simulink library "carterlib"  (R2023a)
settings: Solver=VariableStepAuto  StartTime=0.0  StopTime=10.0  RelTol=1e-3
libraries: arduinolib x6, simulink x1
settings Model: Creator=kawata  LastModifiedBy=kawata
settings RTWCC: GPUComputeCapability=5.0

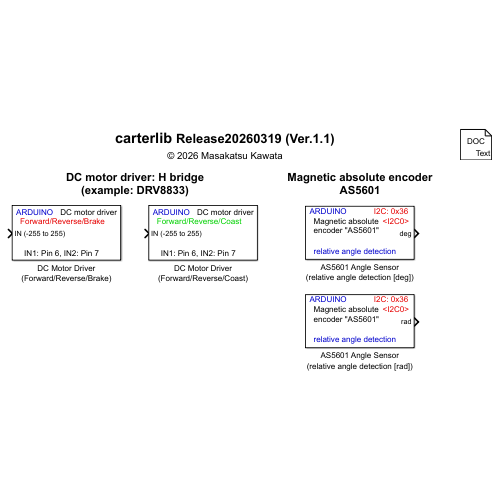
[thumbnail: Simulink's stored preview of the top-level diagram]
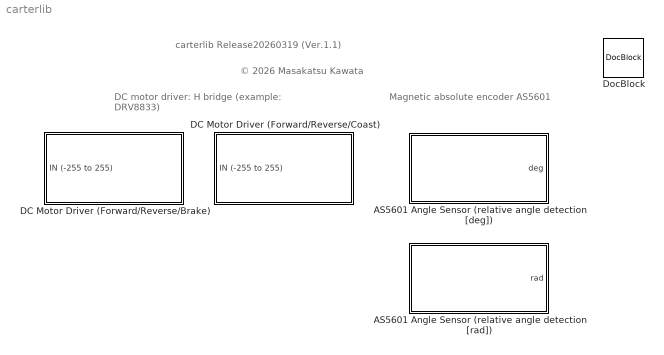
== system carterlib ==
  note: DC motor driver: H bridge
      | (example: DRV8833)
  note: Magnetic absolute encoder
      | AS5601
  note: carterlib Release20260319 (Ver.1.1)
  note: © 2026 Masakatsu Kawata
  AS5601 Angle Sensor (relative angle detection [deg]) : Subsystem  mask{sample_time=-1, I2CModule=0}
      mask prompts: sample_time "Sample Time (-1 for inherited)"; I2CModule "I2C Module"
      mask TypeOptions I2CModule: I2C Read (0x0E: ANGLE)/I2CModule
      mask DialogControl ParameterGroupVar Prompt: パラメーター
      mask Display:
      | color('blue');
      | text(5,60,'ARDUINO')
      | 
      | color('black');
      | text(10,48,'Magnetic absolute')
      | text(10,36,'encoder "AS5601"')
      | 
      | color('blue');
      | text(10, 10, 'relative angle detection');
      | 
      | color('red');
      | text(85, 60, 'I2C: 0x36');
      | 
      | color('red');
      | module = get_param(gcb, 'I2CModule');
      | text(96, 48, ['<I2C' module '>']);
  AS5601 Angle Sensor (relative angle detection [rad]) : Subsystem  mask{sample_time=-1, I2CModule=0}
      mask prompts: sample_time "Sample Time (-1 for inherited)"; I2CModule "I2C Module"
      mask TypeOptions I2CModule: I2C Read (0x0E: ANGLE)/I2CModule
      mask DialogControl ParameterGroupVar Prompt: パラメーター
      mask Display:
      | color('blue');
      | text(5,60,'ARDUINO')
      | 
      | color('black');
      | text(10,48,'Magnetic absolute')
      | text(10,36,'encoder "AS5601"')
      | 
      | color('blue');
      | text(10, 10, 'relative angle detection');
      | 
      | color('red');
      | text(85, 60, 'I2C: 0x36');
      | 
      | color('red');
      | module = get_param(gcb, 'I2CModule');
      | text(96, 48, ['<I2C' module '>']);
  DC Motor Driver (Forward/Reverse/Brake) : Subsystem  mask(Forward/Reverse/Brake){IN1pin=6, IN2pin=7}
      mask prompts: IN1pin "Pin Number (IN1)"; IN2pin "Pin Number (IN2)"
      mask help:
      | IN: -255 to +255
      | ---------------------------------
      | Example
      |
      |   [Arduino MEGA 2560]
      |     Pin Number: 2-13, 44-46
      |
      |   [Arduino UNO R3]
      |     Pin Number: 3, 5, 6, 9-11
      | ---------------------------------
      mask DialogControl ParameterGroupVar Prompt: パラメーター
      mask Display:
      | color('blue');
      | text(5,60,'ARDUINO')
      | 
      | color('black');
      | text(60,60,'DC motor driver')
      | 
      | color('red');
      | text(10,48,['Forward/Reverse/Brake'])
      | 
      | color('black');
      | text(15,8,['IN1: Pin ' num2str(IN1pin) ', IN2: Pin ' num2str(IN2pin)])
  DC Motor Driver (Forward/Reverse/Coast) : Subsystem  mask(Forward/Reverse/Coast){IN1pin=6, IN2pin=7}
      mask prompts: IN1pin "Pin Number (IN1)"; IN2pin "Pin Number (IN2)"
      mask help:
      | IN: -255 to +255
      | ---------------------------------
      | Example
      |
      |   [Arduino MEGA 2560]
      |     Pin Number: 2-13, 44-46
      |
      |   [Arduino UNO R3]
      |     Pin Number: 3, 5, 6, 9-11
      | ---------------------------------
      mask DialogControl ParameterGroupVar Prompt: パラメーター
      mask Display:
      | color('blue');
      | text(5,60,'ARDUINO')
      | 
      | color('black');
      | text(60,60,'DC motor driver')
      | 
      | color('green');
      | text(10,48,'Forward/Reverse/Coast')
      | 
      | color('black');
      | text(15,8,['IN1: Pin ' num2str(IN1pin) ...
      |          ', IN2: Pin ' num2str(IN2pin)])
  DocBlock : simulink/Model-Wide Utilities/DocBlock  DocumentType=Text
      content=|
      | carterlib Ver.1.0
      | Copyright (c) 2026 Masakatsu Kawata
      | Released under the MIT License.
      | See LICENSE for details.

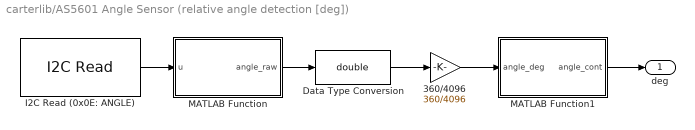
== system carterlib/AS5601 Angle Sensor (relative angle detection [deg]) ==
  360/4096 : Gain  Gain=360/4096
  Data Type Conversion : DataTypeConversion  OutDataTypeStr=double  SaturateOnIntegerOverflow=off  RndMeth=Floor
  I2C Read (0x0E: ANGLE) : arduinolib/I2C Read  I2CModule=0  Mode=Master  SlaveAddress=0x36  SlaveByteOrder=LittleEndian  Direction=Receiver  RegisterAddressMode=on  RegisterAddress=0x0E  SlaveDataType=uint8  DataLength=2  NoAck=off  RepeatedStart=off  OutputStatus=off  blockPlatform=ARDUINO  SampleTime=sample_time
  MATLAB Function : MATLAB Function  TreatAsAtomicUnit=on
  MATLAB Function1 : MATLAB Function  TreatAsAtomicUnit=on
  deg : Outport
  wires:
  MATLAB Function/1(angle_raw) -> Data Type Conversion/1
  360/4096/1 -> MATLAB Function1/1(angle_deg)
  I2C Read (0x0E: ANGLE)/1 -> MATLAB Function/1(u)
  Data Type Conversion/1 -> 360/4096/1
  MATLAB Function1/1(angle_cont) -> deg/1

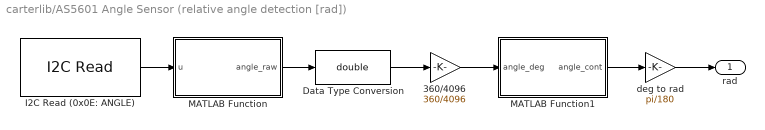
== system carterlib/AS5601 Angle Sensor (relative angle detection [rad]) ==
  360/4096 : Gain  Gain=360/4096
  Data Type Conversion : DataTypeConversion  OutDataTypeStr=double  SaturateOnIntegerOverflow=off  RndMeth=Floor
  I2C Read (0x0E: ANGLE) : arduinolib/I2C Read  I2CModule=0  Mode=Master  SlaveAddress=0x36  SlaveByteOrder=LittleEndian  Direction=Receiver  RegisterAddressMode=on  RegisterAddress=0x0E  SlaveDataType=uint8  DataLength=2  NoAck=off  RepeatedStart=off  OutputStatus=off  blockPlatform=ARDUINO  SampleTime=sample_time
  MATLAB Function : MATLAB Function  TreatAsAtomicUnit=on
  MATLAB Function1 : MATLAB Function  TreatAsAtomicUnit=on
  deg to rad : Gain  Gain=pi/180
  rad : Outport
  wires:
  MATLAB Function1/1(angle_cont) -> deg to rad/1
  Data Type Conversion/1 -> 360/4096/1
  I2C Read (0x0E: ANGLE)/1 -> MATLAB Function/1(u)
  360/4096/1 -> MATLAB Function1/1(angle_deg)
  MATLAB Function/1(angle_raw) -> Data Type Conversion/1
  deg to rad/1 -> rad/1

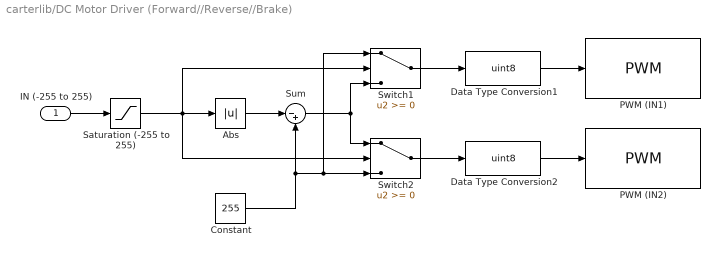
== system carterlib/DC Motor Driver (Forward//Reverse//Brake) ==
  IN (-255 to 255) : Inport
  Abs : Abs  SaturateOnIntegerOverflow=off
  Constant : Constant  Value=255  SampleTime=-1
  Data Type Conversion1 : DataTypeConversion  OutDataTypeStr=uint8  SaturateOnIntegerOverflow=off  RndMeth=Floor
  Data Type Conversion2 : DataTypeConversion  OutDataTypeStr=uint8  SaturateOnIntegerOverflow=off  RndMeth=Floor
  PWM (IN1) : arduinolib/PWM  pinNumber=IN1pin  frequencyType=Default  desiredFrequency=490.2  achievableFrequency=490.2
  PWM (IN2) : arduinolib/PWM  pinNumber=IN2pin  frequencyType=Default  desiredFrequency=490.2  achievableFrequency=490.2
  Saturation (-255 to 255) : Saturate  UpperLimit=255  LowerLimit=-255
  Sum : Sum  Inputs=|-+
  Switch1 : Switch  SaturateOnIntegerOverflow=off  InputSameDT=off
  Switch2 : Switch  SaturateOnIntegerOverflow=off  InputSameDT=off
  wires:
  Data Type Conversion2/1 -> PWM (IN2)/1
  Sum/1 -> Switch1/3, Switch2/1
  Data Type Conversion1/1 -> PWM (IN1)/1
  Constant/1 -> Switch2/3, Switch1/1, Sum/2
  Switch1/1 -> Data Type Conversion1/1
  Abs/1 -> Sum/1
  Switch2/1 -> Data Type Conversion2/1
  Saturation (-255 to 255)/1 -> Switch2/2, Switch1/2, Abs/1
  IN (-255 to 255)/1 -> Saturation (-255 to 255)/1

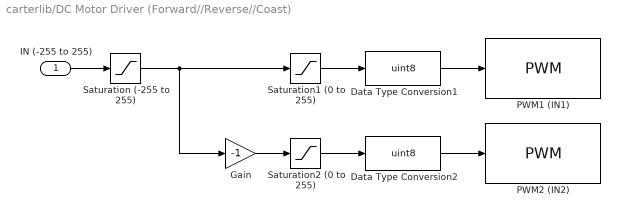
== system carterlib/DC Motor Driver (Forward//Reverse//Coast) ==
  IN (-255 to 255) : Inport
  Data Type Conversion1 : DataTypeConversion  OutDataTypeStr=uint8  SaturateOnIntegerOverflow=off  RndMeth=Floor
  Data Type Conversion2 : DataTypeConversion  OutDataTypeStr=uint8  SaturateOnIntegerOverflow=off  RndMeth=Floor
  Gain : Gain  Gain=-1
  PWM1 (IN1) : arduinolib/PWM  pinNumber=44  frequencyType=Default  desiredFrequency=490.2  achievableFrequency=490.2
  PWM2 (IN2) : arduinolib/PWM  pinNumber=45  frequencyType=Default  desiredFrequency=490.2  achievableFrequency=490.2
  Saturation (-255 to 255) : Saturate  UpperLimit=255  LowerLimit=-255
  Saturation1 (0 to 255) : Saturate  UpperLimit=255  LowerLimit=0
  Saturation2 (0 to 255) : Saturate  UpperLimit=255  LowerLimit=0
  wires:
  IN (-255 to 255)/1 -> Saturation (-255 to 255)/1
  Data Type Conversion2/1 -> PWM2 (IN2)/1
  Gain/1 -> Saturation2 (0 to 255)/1
  Data Type Conversion1/1 -> PWM1 (IN1)/1
  Saturation1 (0 to 255)/1 -> Data Type Conversion1/1
  Saturation (-255 to 255)/1 -> Gain/1, Saturation1 (0 to 255)/1
  Saturation2 (0 to 255)/1 -> Data Type Conversion2/1

== matlab function carterlib/AS5601 Angle Sensor (relative angle detection [deg])/MATLAB Function ==
  data: u input; angle_raw output
function angle_raw = bytes_to_uint12(u)
%#codegen
% u: [MSB LSB] (uint8ベクトル)
raw = bitshift(uint16(u(1)), 8) + uint16(u(2));
angle_raw = bitand(raw, uint16(4095)); % 下位12bitのみ有効

== matlab function carterlib/AS5601 Angle Sensor (relative angle detection [rad])/MATLAB Function ==
  data: u input; angle_raw output
function angle_raw = bytes_to_uint12(u)
%#codegen
% u: [MSB LSB] (uint8ベクトル)
raw = bitshift(uint16(u(1)), 8) + uint16(u(2));
angle_raw = bitand(raw, uint16(4095)); % 下位12bitのみ有効

== matlab function carterlib/AS5601 Angle Sensor (relative angle detection [rad])/MATLAB Function1 ==
  data: angle_deg input; angle_cont output
function angle_cont = unwrap_angle(angle_deg)
persistent prev_angle total_angle
if isempty(prev_angle)
    prev_angle = angle_deg;
    total_angle = 0;
end

diff = angle_deg - prev_angle;
if diff > 180
    diff = diff - 360;
elseif diff < -180
    diff = diff + 360;
end

total_angle = total_angle + diff;
prev_angle = angle_deg;
angle_cont = total_angle;

== matlab function carterlib/AS5601 Angle Sensor (relative angle detection [deg])/MATLAB Function1 ==
  data: angle_deg input; angle_cont output
function angle_cont = unwrap_angle(angle_deg)
persistent prev_angle total_angle
if isempty(prev_angle)
    prev_angle = angle_deg;
    total_angle = 0;
end

diff = angle_deg - prev_angle;
if diff > 180
    diff = diff - 360;
elseif diff < -180
    diff = diff + 360;
end

total_angle = total_angle + diff;
prev_angle = angle_deg;
angle_cont = total_angle;
